simulink model "Copy_of_w12"  (R2025a)
settings: Solver=VariableStepAuto  StartTime=0.0  StopTime=2  MaxStep=1e-4  RelTol=1e-3
values from neighbouring files (symbols this model uses):
  B = 0.0001    [main.m]
  J = 0.045    [main.m]
  Kic = Rs*Wcc    (= 1256.63706144)    [main.m]
  Kpc = Lds*Wcc    (= 18.8495559215)    [main.m]
  Lamf = 0.12    [main.m]
  Lds = 30.0e-3    (= 0.03)    [main.m]
  Lqs = 40.0e-3    (= 0.04)    [main.m]
  P = 24    [main.m]
  Rs = 2    [main.m]
undefined symbols (not defined in the file or in its folder): magnitude
settings Model: Creator=moon  LastModifiedBy=moon
settings RTWCC: GPUComputeCapability=3.5

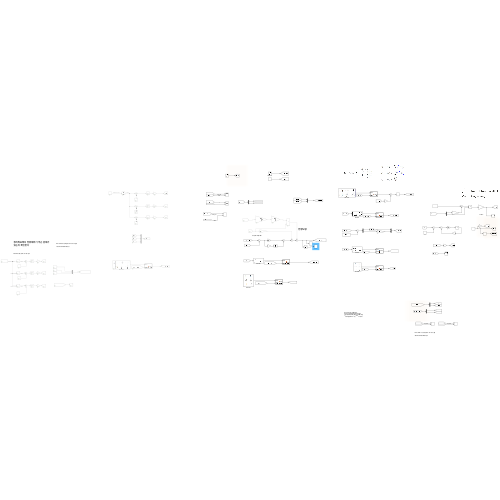
[thumbnail: Simulink's stored preview of the top-level diagram]
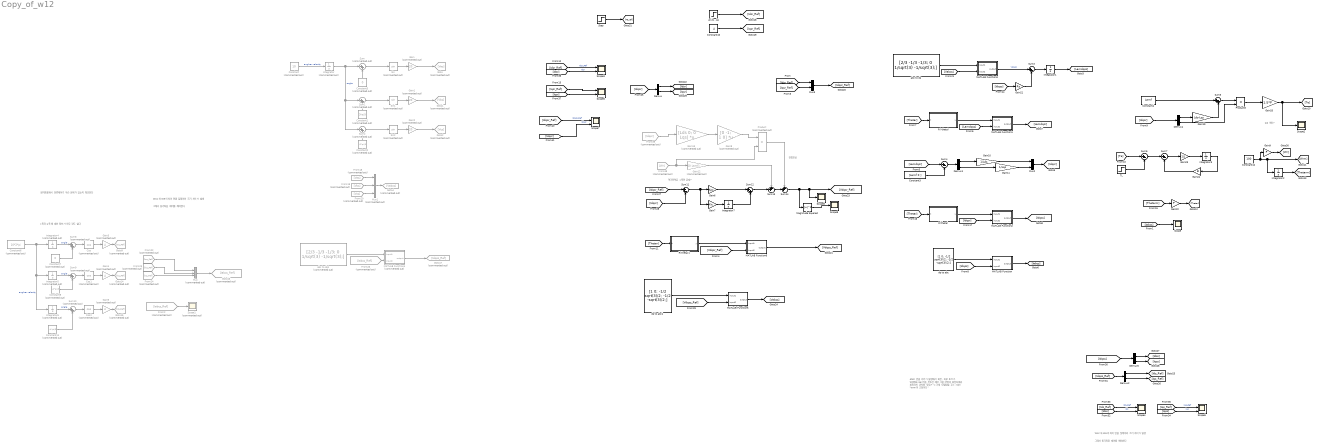
== system Copy_of_w12 ==
  note: 역기전력은 q축만 존재?
  note: 전향보상
  note: 4Nm 만큼 거리가 발생해서 회전,
      | 외부 토크가 발생해도iqs 만큼 무조건 제어
      | 그럼 어떻게 회전자계와 회전자의 위치를 맞춰?
      | -> 기계 모델링을 무시: 대신 "wrm이 고정이다"
  note: d축과 q축 에 대한 정보가 아무 것도 없다
  note: 그래서 동기좌표 제어를 해야한다
  note: Wcc 와 We의 차이 만큼 딜레이와 크기 차이가 발생
  note: 정지좌표에서 전류제어기 무슨 문제가 있는지 확인한다
  note: 1/2 해야?
  note: Wcc 와 We의 차이 만큼 딜레이와 크기 차이가 발생
  note: 그래서 동기좌표 제어를 해야한다
  Constant : Constant  Commented=on  Value=10
  Constant1 : Constant  Commented=on  Value=2*pi/3
  Constant10 : Constant  Value=4
  Constant11 : Constant  Commented=on  Value=-4*pi/3
  Constant12 : Constant  Value=100
  Constant2 : Constant  Commented=on  Value=-2*pi/3
  Constant3 : Constant  Value=[Lamf 0 ]
  Constant4 : Constant  Value=Lamf
  Constant5 : Constant  Commented=on  Value=0
  Constant6 : Constant  Commented=on  Value=10*2*pi
  Constant7 : Constant  Commented=on  Value=0
  Constant9 : Constant  Commented=on  Value=-2*pi/3
  Cos : Trigonometry  Commented=on  Operator=cos
  Cos1 : Trigonometry  Commented=on  Operator=cos
  Cos2 : Trigonometry  Commented=on  Operator=cos
  Demux{,1..2,4..5} (5 alike) : Demux  Outputs=2
  From18 : From  Commented=on  GotoTag=Vas
  From19 : From  Commented=on  GotoTag=Vbs
  From2 : From  Commented=on  GotoTag=Iabcs_Ref
  From20 : From  Commented=on  GotoTag=Vcs
  From22 : From  Commented=on  GotoTag=Ias_Ref
  From23 : From  Commented=on  GotoTag=Ibs_Ref
  From24 : From  Commented=on  GotoTag=Ics_Ref
  From26 : From  Commented=on  GotoTag=Iabcs_Ref
  From38 : From  Commented=on  GotoTag=Wr
  From39 : From  Commented=on  GotoTag=Idqsr
  Gain : Gain  Commented=on  Gain=20
  Gain1 : Gain  Commented=on  Gain=20
  Gain10 : Gain  Gain=1/Lds
  Gain11 : Gain  Gain=1/Lqs
  Gain12 : Gain  Commented=on  Gain=[0 Lamf]
  Gain13 : Gain  Commented=on  Gain=[Lds 0; 0 Lqs]  Multiplication=Matrix(K*u)
  Gain19 : Gain  Gain=Lds-Lqs
  Gain2 : Gain  Commented=on  Gain=20
  Gain20 : Gain  Gain=1.5*P
  Gain21 : Gain  Gain=Rs
  Gain22 : Gain  Gain=P
  Gain23 : Gain  Gain=1/J
  Gain24 : Gain  Gain=B
  Gain3 : Gain  Commented=on  Gain=4
  Gain4 : Gain  Commented=on  Gain=4
  Gain5 : Gain  Commented=on  Gain=4
  Gain6 : Gain  Gain=Kpc
  Gain7 : Gain  Gain=Kic
  Gain8 : Gain  Commented=on  Gain=[0 -1; 1 0]  Multiplication=Matrix(K*u)
  Gain9 : Gain  Gain=P
  Goto : Goto  Commented=on  GotoTag=Vas
  Goto1 : Goto  Commented=on  GotoTag=Vbs
  Goto14 : Goto  Commented=on  GotoTag=Ibs_Ref
  Goto15 : Goto  Commented=on  GotoTag=Ics_Ref
  Goto16 : Goto  Commented=on  GotoTag=Iabcs_Ref
  Goto17 : Goto  Commented=on  GotoTag=Idqss_Ref
  Goto2 : Goto  Commented=on  GotoTag=Vcs
  Goto4 : Goto  Commented=on  GotoTag=Vabcs
  Goto9 : Goto  Commented=on  GotoTag=Ias_Ref
  Integrator{,4..6} (4 alike) : Integrator  Commented=on
  Integrator{1..3,7} (4 alike) : Integrator
  MATLAB Function : MATLAB Function  TreatAsAtomicUnit=on
  MATLAB Function1 : MATLAB Function  TreatAsAtomicUnit=on
  MATLAB Function2 : MATLAB Function  TreatAsAtomicUnit=on
  MATLAB Function3 : MATLAB Function  TreatAsAtomicUnit=on
  MATLAB Function4 : MATLAB Function  Commented=on  TreatAsAtomicUnit=on
  MATLAB Function5 : MATLAB Function  TreatAsAtomicUnit=on
  MATLAB Function6 : MATLAB Function  TreatAsAtomicUnit=on
  Magnitude Squared : Math  Operator=magnitude^2
  Mux : Mux  Commented=on  Inputs=3
  Mux1 : Mux  Commented=on  Inputs=3
  Mux2 : Mux  Inputs=2
  Mux3 : Mux  Inputs=2
  Product : Product  Commented=on
  Product8 : Product
  R(-theta) : Subsystem
      mask Display: image(imread('img/rotateInverseMatrix.png'))
  R(theta) : Subsystem
      mask Display: image(imread('img/rotateMatrix.png'))
  R(theta)1 : Subsystem
      mask Display: image(imread('img/rotateMatrix.png'))
  Scope{,2,8..9} (4 alike) : Scope
      Scope settings: ActiveDisplayYMinimum=-5.1349  ActiveDisplayYMaximum=5.16935
      Scope2 settings: ActiveDisplayYMinimum=-54.40151  ActiveDisplayYMaximum=53.3835  DataLoggingVariableName=ScopeData2
      Scope8 settings: ActiveDisplayYMinimum=-736.65005599169956  ActiveDisplayYMaximum=706.83801315665869
      Scope9 settings: ActiveDisplayYMinimum=-43852.575754075304  ActiveDisplayYMaximum=394673.36359268951  DataLoggingVariableName=ScopeData7
  Scope1 : Scope  Commented=on
      settings: ActiveDisplayYMinimum=-5  ActiveDisplayYMaximum=5
  Scope{3..7} (5 alike) : Scope  NumInputPorts=2
      Scope3 settings: ActiveDisplayYMinimum=-5.21787  ActiveDisplayYMaximum=6.96079  DataLoggingVariableName=ScopeData4
      Scope4 settings: ActiveDisplayYMinimum=-5.10751  ActiveDisplayYMaximum=5.1663  DataLoggingVariableName=ScopeData2
      Scope5 settings: ActiveDisplayYMinimum=-5.08231  ActiveDisplayYMaximum=5.15483  DataLoggingVariableName=ScopeData3
      Scope6 settings: ActiveDisplayYMinimum=-2.15748  ActiveDisplayYMaximum=6.91066  DataLoggingVariableName=ScopeData5
      Scope7 settings: ActiveDisplayYMinimum=-5.25048  ActiveDisplayYMaximum=7.25433  DataLoggingVariableName=ScopeData6
  Sin : Trigonometry  Commented=on
  Sin1 : Trigonometry  Commented=on
  Sin2 : Trigonometry  Commented=on
  Step : Step  Time=0  After=40  SampleTime=0
  Sum{,1..2,8..10} (6 alike) : Sum  Commented=on  Inputs=|++
  Sum{3..4,6..7,11} (5 alike) : Sum  Inputs=|+-
  Sum12 : Sum  Inputs=|++
  Sum13 : Sum  Inputs=++|
  Sum14 : Sum  Inputs=++|
  Sum5 : Sum  Inputs=|++
  TL : Step  Time=0.5  After=4  SampleTime=0
  abc to dq : Constant  Value=[2/3 -1/3 -1/3; 0 1/sqrt(3) -1/sqrt(3);]
      mask Display: image(imread('img/abc2dq.png'))
  abc to dq1 : Constant  Commented=on  Value=[2/3 -1/3 -1/3; 0 1/sqrt(3) -1/sqrt(3);]
      mask Display: image(imread('img/abc2dq.png'))
  "at 2s , 4A" : Step  Time=2  After=4  SampleTime=0
  dq to abc : Constant  Value=[1 0; -1/2 sqrt(3)/2; -1/2 -sqrt(3)/2;]
      mask Display: image(imread('img/dq2abc.png'))
  dq to abc1 : Constant  Value=[1 0; -1/2 sqrt(3)/2; -1/2 -sqrt(3)/2;]
      mask Display: image(imread('img/dq2abc.png'))
  wires:
  Gain/1 -> Goto/1
  Sin/1 -> Gain/1
  Sum/1 -> Sin/1
  Constant/1 -> Integrator/1  "angluar velocity"
  Sin1/1 -> Gain1/1
  Gain1/1 -> Goto1/1
  Sum1/1 -> Sin1/1
  Gain2/1 -> Goto2/1
  Sum2/1 -> Sin2/1
  Sin2/1 -> Gain2/1
  Integrator/1 -> Sum2/1, Sum1/1, Sum/1  "angle"
  Constant1/1 -> Sum1/2
  Constant2/1 -> Sum2/2
  Sum3/1 -> Integrator1/1
  Integrator1/1 -> [Lamdqss]
  MATLAB Function3/1(output) -> Sum3/1  "Vdqss"
  [Lamdqsr] -> Sum4/1
  Constant3/1 -> Sum4/2
  Sum4/1 -> Demux1/1
  Demux1/1 -> Gain10/1
  Demux1/2 -> Gain11/1
  Gain10/1 -> Mux2/1
  Gain11/1 -> Mux2/2
  Mux2/1 -> [Idqsr]
  [Idqsr] -> Demux4/1
  Demux4/1 -> Gain19/1
  Constant4/1 -> Sum5/1
  Gain19/1 -> Sum5/2
  Sum5/1 -> Product8/1
  Demux4/2 -> Product8/2
  Product8/1 -> Gain20/1
  Gain20/1 -> Scope2/1, [Te]
  [Te] -> Sum6/1
  Sum6/1 -> Sum7/1
  Integrator3/1 -> Gain24/1
  TL/1 -> Sum6/2
  [Idqss] -> Gain21/1
  Gain21/1 -> Sum3/2
  Gain22/1 -> [Thetar]
  [Thetarm] -> Gain22/1
  Integrator2/1 -> [Thetarm]
  Sum7/1 -> Gain23/1
  Gain23/1 -> Integrator3/1
  Gain24/1 -> Sum7/2
  dq to abc/1 -> MATLAB Function/1(input1)
  [Idqss] -> MATLAB Function/2(input2)
  MATLAB Function/1(output) -> [Iabcs]
  [Lamdqss] -> MATLAB Function1/2(input2)
  MATLAB Function1/1(output) -> [Lamdqsr]
  [Thetar] -> R(-theta)/1(t)
  R(-theta)/1(y) -> MATLAB Function1/1(input1)
  MATLAB Function2/1(output) -> [Idqss]
  [Thetar] -> R(theta)/1(t)
  R(theta)/1(y) -> MATLAB Function2/1(input1)
  [Idqsr] -> MATLAB Function2/2(input2)
  abc to dq/1 -> MATLAB Function3/1(input1)
  [Vabcs] -> MATLAB Function3/2(input2)
  From18/1 -> Mux1/1
  From19/1 -> Mux1/2
  From20/1 -> Mux1/3
  Mux1/1 -> Goto4/1
  Constant12/1 -> Gain9/1, Integrator2/1, [Wrm]
  [Iabcs] -> Scope/1
  Constant5/1 -> Sum/2
  Cos/1 -> Gain3/1
  Integrator4/1 -> Sum8/1  "angle"
  Constant7/1 -> Sum8/2
  Sum8/1 -> Cos/1
  Gain3/1 -> Goto9/1
  Gain4/1 -> Goto14/1
  Constant9/1 -> Sum9/2
  Integrator5/1 -> Sum9/1  "angle"
  Sum9/1 -> Cos1/1
  Cos1/1 -> Gain4/1
  Gain5/1 -> Goto15/1
  Constant11/1 -> Sum10/2
  Integrator6/1 -> Sum10/1  "angle"
  Sum10/1 -> Cos2/1
  Cos2/1 -> Gain5/1
  Constant6/1 -> Integrator6/1, Integrator5/1, Integrator4/1  "angluar velocity"
  From22/1 -> Mux/1
  From23/1 -> Mux/2
  From24/1 -> Mux/3
  Mux/1 -> Goto16/1
  MATLAB Function4/1(output) -> Goto17/1
  abc to dq1/1 -> MATLAB Function4/1(input1)
  From26/1 -> MATLAB Function4/2(input2)
  [Idqsr_Ref] -> Sum11/1
  Gain6/1 -> Sum12/1
  Sum11/1 -> Gain7/1, Gain6/1
  Gain7/1 -> Integrator7/1
  Integrator7/1 -> Sum12/2
  [Idqsr] -> Sum11/2
  dq to abc1/1 -> MATLAB Function5/1(input1)
  MATLAB Function5/1(output) -> [Vabcs]
  [Vdqss_Ref] -> MATLAB Function5/2(input2)
  Demux2/2 -> [Iqs_Ref]
  Demux2/1 -> [Ids_Ref]
  [Idqss_Ref] -> Demux2/1
  [Idqss] -> Demux5/1
  Demux5/1 -> [Idss]
  Demux5/2 -> [Iqss]
  [Ids_Ref] -> Scope4/1  "Ids_Ref"
  [Idss] -> Scope4/2  "Ids"
  [Iqss] -> Scope5/2  "Iqs"
  [Iqs_Ref] -> Scope5/1  "Iqs_Ref"
  From2/1 -> Scope1/1
  "at 2s , 4A"/1 -> [Idsr_Ref]
  Constant10/1 -> [Iqsr_Ref]
  [Iqsr_Ref] -> Mux3/2
  [Idsr_Ref] -> Mux3/1
  Mux3/1 -> [Idqsr_Ref]
  MATLAB Function6/1(output) -> [Vdqss_Ref]
  R(theta)1/1(y) -> MATLAB Function6/1(input1)
  [Vdqsr_Ref] -> MATLAB Function6/2(input2)
  [Thetar] -> R(theta)1/1(t)
  [Idqsr] -> Demux/1
  Demux/2 -> [Iqsr]
  Demux/1 -> [Idsr]
  [Idsr_Ref] -> Scope3/1  "Idsr_Ref"
  [Idsr] -> Scope3/2  "Idsr"
  [Iqsr] -> Scope6/2
  [Iqsr_Ref] -> Scope6/1
  Sum12/1 -> Sum13/2
  Gain9/1 -> [Wr]
  From38/1 -> Product/2, Gain12/1
  Gain12/1 -> Sum13/1
  Sum13/1 -> Sum14/2
  From39/1 -> Gain13/1
  Gain13/1 -> Gain8/1
  Gain8/1 -> Product/1
  Product/1 -> Sum14/1
  [Idqsr_Ref] -> Scope7/1  "Idqsr_Ref"
  [Idqsr] -> Scope7/2  "Idqsr"
  Step/1 -> [Te_ref]
  Magnitude Squared/1 -> Scope9/1
  Sum14/1 -> Magnitude Squared/1, Scope8/1, [Vdqsr_Ref]

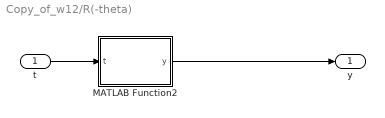
== system Copy_of_w12/R(-theta) ==
  t : Inport
  MATLAB Function2 : MATLAB Function  TreatAsAtomicUnit=on
  y : Outport
  wires:
  MATLAB Function2/1(y) -> y/1
  t/1 -> MATLAB Function2/1(t)

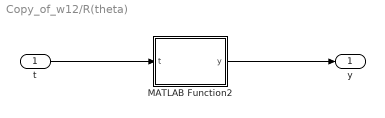
== system Copy_of_w12/R(theta) ==
  t : Inport
  MATLAB Function2 : MATLAB Function  TreatAsAtomicUnit=on
  y : Outport
  wires:
  MATLAB Function2/1(y) -> y/1
  t/1 -> MATLAB Function2/1(t)

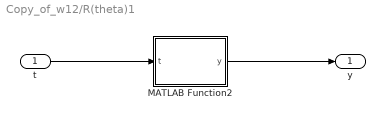
== system Copy_of_w12/R(theta)1 ==
  t : Inport
  MATLAB Function2 : MATLAB Function  TreatAsAtomicUnit=on
  y : Outport
  wires:
  MATLAB Function2/1(y) -> y/1
  t/1 -> MATLAB Function2/1(t)

== matlab function Copy_of_w12/MATLAB Function ==
  data: input1 input; output output; input2 input
function output = matrix_multiply(input1, input2)
    % 행렬 곱셈 (input1의 열 수 = input2의 행 수)
    output = input1 * input2;
end

== matlab function Copy_of_w12/R(-theta)/MATLAB Function2 ==
  data: t input; y output
function y = matrix_output(t)
y = [cos(t) sin(t); -sin(t) cos(t)];

== matlab function Copy_of_w12/MATLAB Function2 ==
  data: input1 input; output output; input2 input
function output = matrix_multiply(input1, input2)
    % 행렬 곱셈 (input1의 열 수 = input2의 행 수)
    output = input1 * input2;
end

== matlab function Copy_of_w12/R(theta)/MATLAB Function2 ==
  data: t input; y output
function y = matrix_output(t)
y = [cos(t) -sin(t); sin(t) cos(t)];

== matlab function Copy_of_w12/MATLAB Function3 ==
  data: input1 input; output output; input2 input
function output = matrix_multiply(input1, input2)
    % 행렬 곱셈 (input1의 열 수 = input2의 행 수)
    output = input1 * input2;
end

== matlab function Copy_of_w12/MATLAB Function4 ==
  data: input1 input; output output; input2 input
function output = matrix_multiply(input1, input2)
    % 행렬 곱셈 (input1의 열 수 = input2의 행 수)
    output = input1 * input2;
end

== matlab function Copy_of_w12/MATLAB Function5 ==
  data: input1 input; output output; input2 input
function output = matrix_multiply(input1, input2)
    % 행렬 곱셈 (input1의 열 수 = input2의 행 수)
    output = input1 * input2;
end

== matlab function Copy_of_w12/MATLAB Function6 ==
  data: input1 input; output output; input2 input
function output = matrix_multiply(input1, input2)
    % 행렬 곱셈 (input1의 열 수 = input2의 행 수)
    output = input1 * input2;
end

== matlab function Copy_of_w12/R(theta)1/MATLAB Function2 ==
  data: t input; y output
function y = matrix_output(t)
y = [cos(t) -sin(t); sin(t) cos(t)];

== matlab function Copy_of_w12/MATLAB Function1 ==
  data: input1 input; output output; input2 input
function output = matrix_multiply(input1, input2)
    % 행렬 곱셈 (input1의 열 수 = input2의 행 수)
    output = input1 * input2;
end
